simulink model "WDS_random"  (R2021a)
settings: Solver=FixedStepDiscrete  StartTime=0.0  StopTime=T_final  FixedStep=T_sample  RelTol=1e-3
values from neighbouring files (symbols this model uses):
  I_attack = sort(I_attack)    [prepare_random_dataset.m]
  I_attack_local = randperm(n_meas,n_attack)    [prepare_random_dataset.m]
  n_attack = nn_attack(iter)    [prepare_random_dataset.m]
undefined symbols (not defined in the file or in its folder): A_bar_d, B_bar_d, C_obsv_d, Cm, D_obsv_d, H0, H0_perp, H1, K, Lu, Ly, n_int, n_meas, offset, T, T_sample, T_start_attack, T_start_opt, U0, x0, xd, Y0
libraries: simulink x6
settings Model: Creator=Abelb  LastModifiedBy=Abelb

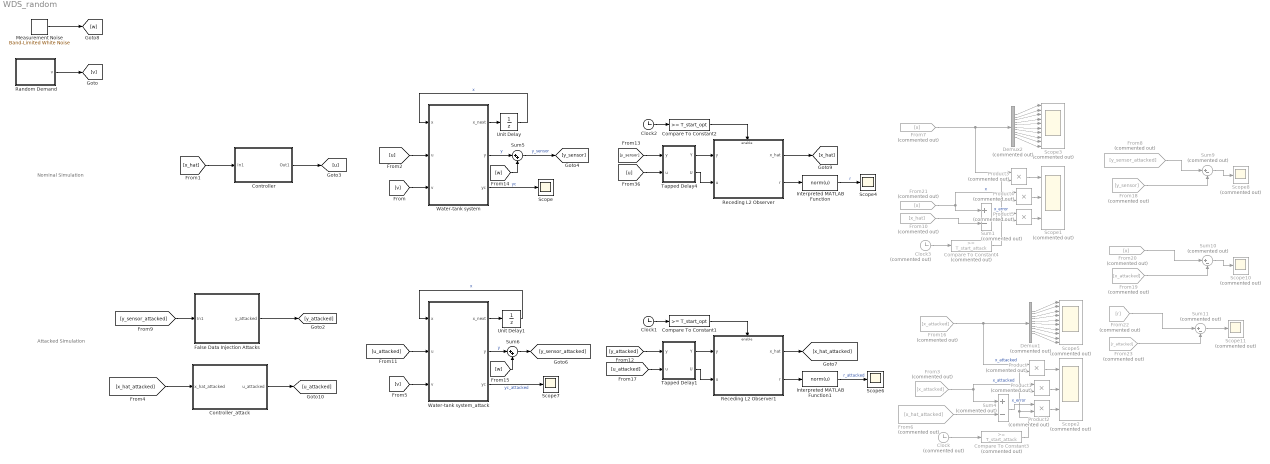
== system WDS_random ==
  note: Nominal Simulation
  note: Attacked Simulation
  Clock : Clock  Commented=on
  Clock1 : Clock
  Clock2 : Clock
  Clock3 : Clock  Commented=on
  Compare To Constant1 : simulink/Logic and Bit Operations/Compare To Constant  relop=>=  const=T_start_opt  OutDataTypeStr=boolean
  Compare To Constant2 : simulink/Logic and Bit Operations/Compare To Constant  relop=>=  const=T_start_opt  OutDataTypeStr=boolean
  Compare To Constant3 : simulink/Logic and Bit Operations/Compare To Constant  Commented=on  relop=>=  const=T_start_attack  OutDataTypeStr=boolean
  Compare To Constant4 : simulink/Logic and Bit Operations/Compare To Constant  Commented=on  relop=>=  const=T_start_attack  OutDataTypeStr=boolean
  Controller : Subsystem
  Controller_attack : Subsystem
  Demux1 : Demux  Commented=on  Outputs=n_states
  Demux2 : Demux  Commented=on  Outputs=n_states
  False Data Injection Attacks : Subsystem
  From10 : From  Commented=on  GotoTag=x_hat
  From16 : From  Commented=on  GotoTag=x_attacked
  From18 : From  Commented=on  GotoTag=y_sensor
  From19 : From  Commented=on  GotoTag=x_attacked
  From20 : From  Commented=on  GotoTag=x
  From21 : From  Commented=on  GotoTag=x
  From22 : From  Commented=on  GotoTag=r
  From23 : From  Commented=on  GotoTag=r_attacked
  From3 : From  Commented=on  GotoTag=x_attacked
  From6 : From  Commented=on  GotoTag=x_hat_attacked
  From7 : From  Commented=on  GotoTag=x
  From8 : From  Commented=on  GotoTag=y_sensor_attacked
  Interpreted MATLAB Function : MATLABFcn  MATLABFcn=norm(u)
  Interpreted MATLAB Function1 : MATLABFcn  MATLABFcn=norm(u)
  Measurement Noise : simulink/Sources/Band-Limited White Noise  Cov=[0.001]  Ts=T_sample  seed=[23341]
  Product{,1..5} (6 alike) : Product  Commented=on
  Random Demand : Subsystem
  Receding L2 Observer : Subsystem
  Receding L2 Observer1 : Subsystem
  Scope{,4,6..7} (4 alike) : Scope
  Scope1 : Scope  Commented=on  NumInputPorts=3
  Scope10 : Scope  Commented=on
  Scope11 : Scope  Commented=on
  Scope2 : Scope  Commented=on  NumInputPorts=3
  Scope3 : Scope  Commented=on  NumInputPorts=10
  Scope5 : Scope  Commented=on  NumInputPorts=10
  Scope8 : Scope  Commented=on
  Sum1 : Sum  Commented=on  Inputs=+-
  Sum10 : Sum  Commented=on  Inputs=|+-
  Sum11 : Sum  Commented=on  Inputs=|+-
  Sum4 : Sum  Commented=on  Inputs=+-
  Sum5 : Sum  Inputs=|++
  Sum6 : Sum  Inputs=|++
  Sum9 : Sum  Commented=on  Inputs=|+-
  Tapped Delay1 : Subsystem
  Tapped Delay4 : Subsystem
  Unit Delay : UnitDelay  InitialCondition=x0  SampleTime=-1  HasFrameUpgradeWarning=on
  Unit Delay1 : UnitDelay  InitialCondition=x0  SampleTime=-1  HasFrameUpgradeWarning=on
  Water-tank system : MATLAB Function  TreatAsAtomicUnit=on
  Water-tank system_attack : MATLAB Function  TreatAsAtomicUnit=on
  wires:
  Unit Delay/1 -> Water-tank system/1(x)  "x"
  Water-tank system/1(x_next) -> Unit Delay/1
  [u] -> Water-tank system/2(u)
  Tapped Delay4/2(U) -> Receding L2 Observer/2(u)
  Receding L2 Observer/1(x_hat) -> [x_hat]
  [u] -> Tapped Delay4/2(u)
  Compare To Constant2/1 -> Receding L2 Observer/Enable
  Tapped Delay4/1(Y) -> Receding L2 Observer/1(y)
  Clock2/1 -> Compare To Constant2/1
  Demux2/4 -> Scope3/4
  Demux2/3 -> Scope3/3
  Demux2/5 -> Scope3/5
  Demux2/9 -> Scope3/9
  Demux2/10 -> Scope3/10
  Demux2/7 -> Scope3/7
  Demux2/1 -> Scope3/1
  Demux2/6 -> Scope3/6
  Demux2/2 -> Scope3/2
  Demux2/8 -> Scope3/8
  [y_sensor] -> Tapped Delay4/1(y)
  Sum5/1 -> [y_sensor]  "y_sensor"
  Water-tank system/2(y) -> Sum5/1  "y"
  Random Demand/1(v) -> [v]
  [v] -> Water-tank system/3(v)
  Interpreted MATLAB Function/1 -> Scope4/1  "r"
  Receding L2 Observer/2(r) -> Interpreted MATLAB Function/1
  Water-tank system_attack/2(y) -> Sum6/1  "y"
  [v] -> Water-tank system_attack/3(v)
  Receding L2 Observer1/2(r) -> Interpreted MATLAB Function1/1
  Interpreted MATLAB Function1/1 -> Scope6/1  "r_attacked"
  Unit Delay1/1 -> Water-tank system_attack/1(x)  "x"
  Tapped Delay1/1(Y) -> Receding L2 Observer1/1(y)
  Demux1/9 -> Scope5/9
  From6/1 -> Sum4/2
  Demux1/7 -> Scope5/7
  Sum6/1 -> [y_sensor_attacked]
  Demux1/8 -> Scope5/8
  From16/1 -> Product/1, Demux1/1  "x_attacked"
  [u_attacked] -> Water-tank system_attack/2(u)
  Demux1/6 -> Scope5/6
  Demux1/4 -> Scope5/4
  Demux1/1 -> Scope5/1
  [y_attacked] -> Tapped Delay1/1(y)
  [u_attacked] -> Tapped Delay1/2(u)
  From3/1 -> Sum4/1, Product1/1  "x_attacked"
  Demux1/2 -> Scope5/2
  Demux1/10 -> Scope5/10
  Demux1/5 -> Scope5/5
  Receding L2 Observer1/1(x_hat) -> [x_hat_attacked]
  Demux1/3 -> Scope5/3
  Tapped Delay1/2(U) -> Receding L2 Observer1/2(u)
  Compare To Constant1/1 -> Receding L2 Observer1/Enable
  Clock1/1 -> Compare To Constant1/1
  Water-tank system_attack/1(x_next) -> Unit Delay1/1
  Measurement Noise/1 -> [w]
  [w] -> Sum5/2
  [w] -> Sum6/2
  From8/1 -> Sum9/1
  From18/1 -> Sum9/2
  Sum9/1 -> Scope8/1
  Sum10/1 -> Scope10/1
  From20/1 -> Sum10/1
  From19/1 -> Sum10/2
  Sum11/1 -> Scope11/1
  From23/1 -> Sum11/2
  From22/1 -> Sum11/1
  [x_hat_attacked] -> Controller_attack/1(x_hat_attacked)
  Controller_attack/1(u_attacked) -> [u_attacked]
  [y_sensor_attacked] -> False Data Injection Attacks/1(In1)
  False Data Injection Attacks/1(y_attacked) -> [y_attacked]
  [x_hat] -> Controller/1(In1)
  Controller/1(Out1) -> [u]
  Clock/1 -> Compare To Constant3/1
  Compare To Constant3/1 -> Product2/2, Product1/2, Product/2
  Product/1 -> Scope2/1
  Product1/1 -> Scope2/2
  Product2/1 -> Scope2/3
  Sum4/1 -> Product2/1  "x_error"
  From7/1 -> Product3/1, Demux2/1
  Sum1/1 -> Product5/1  "x_error"
  Product5/1 -> Scope1/3
  Product4/1 -> Scope1/2
  Clock3/1 -> Compare To Constant4/1
  Product3/1 -> Scope1/1
  From21/1 -> Product4/1, Sum1/1  "x"
  From10/1 -> Sum1/2
  Compare To Constant4/1 -> Product5/2, Product4/2, Product3/2
  Water-tank system/3(yc) -> Scope/1  "yc"
  Water-tank system_attack/3(yc) -> Scope7/1  "yc_attacked"

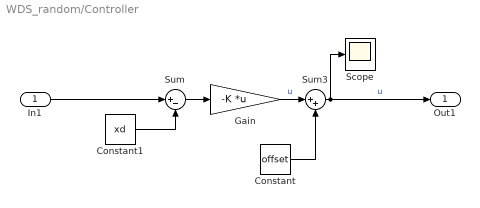
== system WDS_random/Controller ==
  In1 : Inport
  Constant : Constant  Value=offset
  Constant1 : Constant  Value=xd
  Gain : Gain  Gain=-K  Multiplication=Matrix(K*u) (u vector)
  Scope : Scope
  Sum : Sum  Inputs=|+-
  Sum3 : Sum  Inputs=|++
  Out1 : Outport
  wires:
  Sum3/1 -> Out1/1, Scope/1  "u"
  Constant/1 -> Sum3/2
  Constant1/1 -> Sum/2
  Gain/1 -> Sum3/1  "u"
  Sum/1 -> Gain/1
  In1/1 -> Sum/1

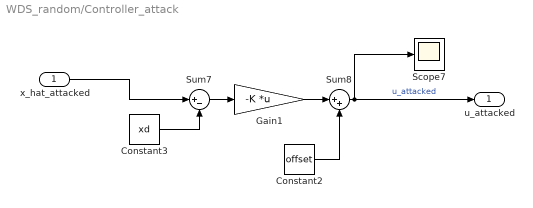
== system WDS_random/Controller_attack ==
  x_hat_attacked : Inport
  Constant2 : Constant  Value=offset
  Constant3 : Constant  Value=xd
  Gain1 : Gain  Gain=-K  Multiplication=Matrix(K*u) (u vector)
  Scope7 : Scope
  Sum7 : Sum  Inputs=|+-
  Sum8 : Sum  Inputs=|++
  u_attacked : Outport
  wires:
  x_hat_attacked/1 -> Sum7/1
  Sum7/1 -> Gain1/1
  Gain1/1 -> Sum8/1
  Constant2/1 -> Sum8/2
  Sum8/1 -> u_attacked/1, Scope7/1  "u_attacked"
  Constant3/1 -> Sum7/2

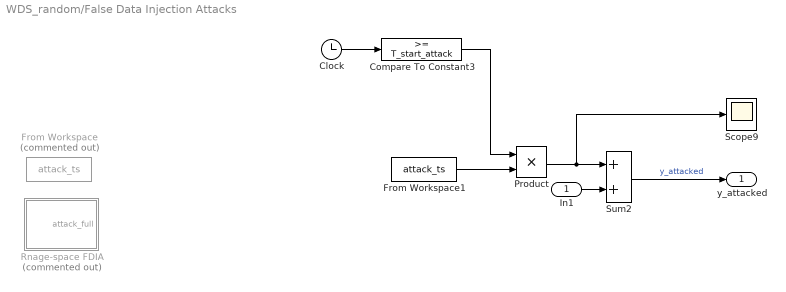
== system WDS_random/False Data Injection Attacks ==
  In1 : Inport
  Clock : Clock
  Compare To Constant3 : simulink/Logic and Bit Operations/Compare To Constant  relop=>=  const=T_start_attack  OutDataTypeStr=boolean
  From Workspace : FromWorkspace  Commented=on  VariableName=attack_ts  SampleTime=T_sample  Interpolate=off  OutputAfterFinalValue=Setting to zero
  From Workspace1 : FromWorkspace  VariableName=attack_ts  SampleTime=T_sample  Interpolate=off  OutputAfterFinalValue=Setting to zero
  Product : Product
  Rnage-space FDIA : MATLAB Function  Commented=on  TreatAsAtomicUnit=on
  Scope9 : Scope
  Sum2 : Sum
  y_attacked : Outport
  wires:
  Compare To Constant3/1 -> Product/1
  In1/1 -> Sum2/2
  Product/1 -> Sum2/1, Scope9/1
  Clock/1 -> Compare To Constant3/1
  Sum2/1 -> y_attacked/1  "y_attacked"
  From Workspace1/1 -> Product/2

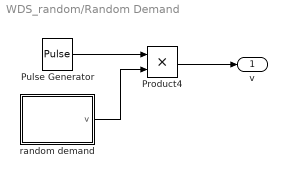
== system WDS_random/Random Demand ==
  " random demand" : MATLAB Function  TreatAsAtomicUnit=on
  Product4 : Product
  Pulse Generator : DiscretePulseGenerator  Period=10  SampleTime=T_sample
  v : Outport
  wires:
  " random demand"/1(v) -> Product4/2
  Product4/1 -> v/1
  Pulse Generator/1 -> Product4/1

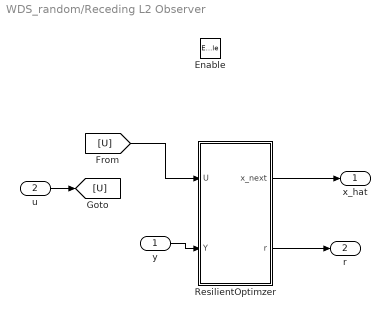
== system WDS_random/Receding L2 Observer ==
  y : Inport
  u : Inport  Port=2
  Enable : EnablePort
  ResilientOptimzer : MATLAB Function  TreatAsAtomicUnit=on
  x_hat : Outport
  r : Outport  Port=2
  wires:
  u/1 -> [U]
  y/1 -> ResilientOptimzer/2(Y)
  [U] -> ResilientOptimzer/1(U)
  ResilientOptimzer/1(x_next) -> x_hat/1
  ResilientOptimzer/2(r) -> r/1

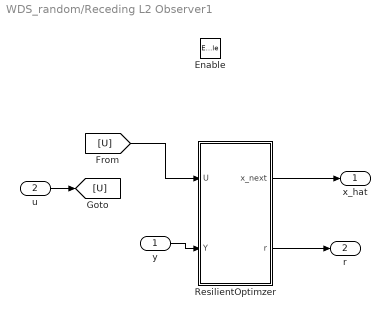
== system WDS_random/Receding L2 Observer1 ==
  y : Inport
  u : Inport  Port=2
  Enable : EnablePort
  ResilientOptimzer : MATLAB Function  TreatAsAtomicUnit=on
  x_hat : Outport
  r : Outport  Port=2
  wires:
  u/1 -> [U]
  y/1 -> ResilientOptimzer/2(Y)
  [U] -> ResilientOptimzer/1(U)
  ResilientOptimzer/1(x_next) -> x_hat/1
  ResilientOptimzer/2(r) -> r/1

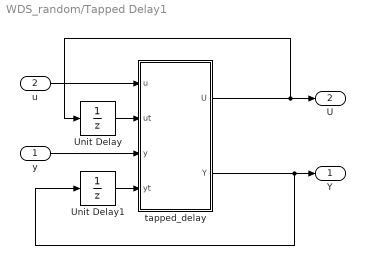
== system WDS_random/Tapped Delay1 ==
  y : Inport
  u : Inport  Port=2
  Unit Delay : UnitDelay  InitialCondition=U0  SampleTime=-1  HasFrameUpgradeWarning=on
  Unit Delay1 : UnitDelay  InitialCondition=Y0  SampleTime=-1  HasFrameUpgradeWarning=on
  tapped_delay : MATLAB Function  TreatAsAtomicUnit=on
  Y : Outport
  U : Outport  Port=2
  wires:
  u/1 -> tapped_delay/1(u)
  y/1 -> tapped_delay/3(y)
  tapped_delay/1(U) -> Unit Delay/1, U/1
  tapped_delay/2(Y) -> Unit Delay1/1, Y/1
  Unit Delay/1 -> tapped_delay/2(ut)
  Unit Delay1/1 -> tapped_delay/4(yt)

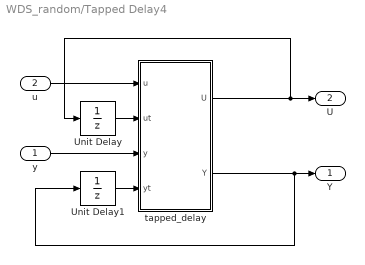
== system WDS_random/Tapped Delay4 ==
  y : Inport
  u : Inport  Port=2
  Unit Delay : UnitDelay  InitialCondition=U0  SampleTime=-1  HasFrameUpgradeWarning=on
  Unit Delay1 : UnitDelay  InitialCondition=Y0  SampleTime=-1  HasFrameUpgradeWarning=on
  tapped_delay : MATLAB Function  TreatAsAtomicUnit=on
  Y : Outport
  U : Outport  Port=2
  wires:
  u/1 -> tapped_delay/1(u)
  y/1 -> tapped_delay/3(y)
  tapped_delay/1(U) -> Unit Delay/1, U/1
  tapped_delay/2(Y) -> Unit Delay1/1, Y/1
  Unit Delay/1 -> tapped_delay/2(ut)
  Unit Delay1/1 -> tapped_delay/4(yt)

== matlab function WDS_random/Tapped Delay4/tapped_delay ==
  data: u input; U output; ut input; y input; yt input; Y output
function [U,Y] = fcn(u,ut,y,yt)
%% tapped_delay_array
% shift columns from tapped matrix to the left and appends most recent
% vector to the last column
%%% input
ut(:,1:end-1) = ut(:,2:end);
ut(:,end) = u;
U = ut;
%%% output
yt(:,1:end-1) = yt(:,2:end);
yt(:,end) = y;
Y = yt;

== matlab function WDS_random/Receding L2 Observer/ResilientOptimzer ==
  data: x_next output; U input; Y input; Ly parameter; Lu parameter; H0_perp parameter; H1 parameter; r output
function [x_next,r]  = fcn(U,Y, Ly, Lu,H0_perp, H1)


u_local = U(:,1:end-1);
% vectorized
u = u_local(:);
y = Y(:);

x_next = zeros(10,1);
x_next(:) = Ly*y + Lu*u;

r = H0_perp*(y-H1*u);

== matlab function WDS_random/Receding L2 Observer1/ResilientOptimzer ==
  data: x_next output; U input; Y input; Ly parameter; Lu parameter; n_int parameter; T parameter; H0_perp parameter; H1 parameter; r output
function [x_next,r]  = fcn(U,Y, Ly, Lu,n_int,T,H0_perp, H1)

u_local = zeros(n_int,T+1-1);
u_local(:,:) = U(:,1:end-1);
% vectorized
u = u_local(:);
y = Y(:);

x_next = zeros(10,1);
x_next(:) = Ly*y + Lu*u;

r = H0_perp*(y-H1*u);

== matlab function WDS_random/False Data Injection Attacks/Rnage-space FDIA ==
  data: attack_full output; H0 parameter; n_meas parameter; I_attack_local parameter; n_attack parameter; I_attack parameter
function attack_full = fcn(H0,n_meas,I_attack_local, n_attack,I_attack)
%% generate FDIA on the range space of T time horizon state-output transfer matrix H0

in =0.3 * rand(size(H0(I_attack),2),1);

eT = H0(I_attack)*in;

e = eT(1:n_attack);

attack_full = zeros(n_meas,1);
for iter = 1:n_attack
    attack_full(I_attack_local(iter)) = e(iter);
end

== matlab function WDS_random/Tapped Delay1/tapped_delay ==
  data: u input; U output; ut input; y input; yt input; Y output
function [U,Y] = fcn(u,ut,y,yt)
%% tapped_delay_array
% shift columns from tapped matrix to the left and appends most recent
% vector to the last column
%%% input
ut(:,1:end-1) = ut(:,2:end);
ut(:,end) = u;
U = ut;
%%% output
yt(:,1:end-1) = yt(:,2:end);
yt(:,end) = y;
Y = yt;

== matlab function WDS_random/Water-tank system_attack ==
  data: x input; x_next output; u input; v input; y output; A_bar_d parameter; C_obsv_d parameter; B_bar_d parameter; D_obsv_d parameter; Cm parameter; yc output
function [x_next,y,yc] = fcn(x,u,v,A_bar_d,C_obsv_d,B_bar_d,D_obsv_d,Cm)
% Discrete state-space model for system

x_next = A_bar_d*x + B_bar_d*u - v;

y = C_obsv_d*x + D_obsv_d*u;

% critical measurements
yc = Cm*x;

== matlab function WDS_random/Random Demand/ random demand ==
  data: v output; n_states parameter
function v = fcn(n_states)

v = 0.3*rand(n_states,1);

== matlab function WDS_random/Water-tank system ==
  data: x input; x_next output; u input; v input; y output; A_bar_d parameter; C_obsv_d parameter; B_bar_d parameter; D_obsv_d parameter; Cm parameter; yc output
function [x_next,y,yc] = fcn(x,u,v,A_bar_d,C_obsv_d,B_bar_d,D_obsv_d,Cm)
% Discrete state-space model for system

x_next = A_bar_d*x + B_bar_d*u - v;

y = C_obsv_d*x + D_obsv_d*u;

% critical measurements
yc = Cm*x;
